simulink model "model1"  (R2024b)
settings: Solver=VariableStepAuto  StartTime=0.0  StopTime=10.0  RelTol=1e-3
values from neighbouring files (symbols this model uses):
  A = [1,2;-3,-4]    [design_AL.m]    (also in run1.m = [[0,1;0,-B/M],zeros(2,2);zeros(2,2),[0,1;0,-Br/J]]; run_p.m; test.m = -1; test2.m = -1)
  Bw = [1;1]    [design_AL.m]    (also in run1.m = zeros(5,1); run_p.m; test.m = 1; test2.m = 1)
  C = [2,1;4,2]    [design_AL.m]    (also in run1.m = [1,0,0,0;0,1,0,0;0,1,0,0;0,0,1,0;0,0,0,1]; run_p.m; test.m = [1;2]; test2.m = [1;2])
  Dw = [1;1]    [design_AL.m]    (also in run1.m = [1;1;1;1;1]; run_p.m; test.m = [1;2]; test2.m = [1;2]*1+[2;-1]*1)
  L = P \ Y    [run_p.m]    (also in test.m = [1,1]; test2.m = inv(P)*Y; test3.m = inv(P)*Y; test4.m = sym('x',[n,p]))
  Lmbda = [x1val,1]    [test2.m]
  Pival = eye(p)-C*pinv(C'*C)*C'    [test.m]    (also in test2.m; test3.m; test4.m)
settings Model: Creator=mehmetcanevi  LastModifiedBy=Mehmet

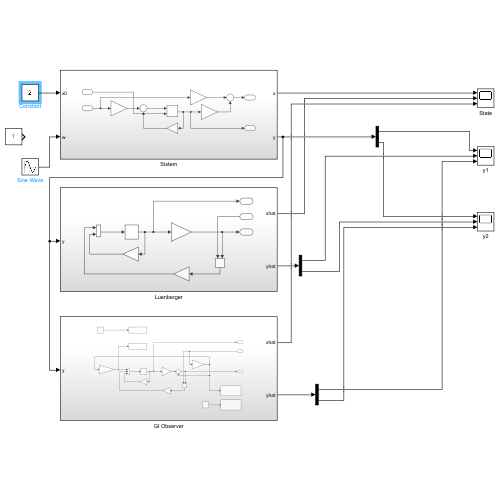
[thumbnail: Simulink's stored preview of the top-level diagram]
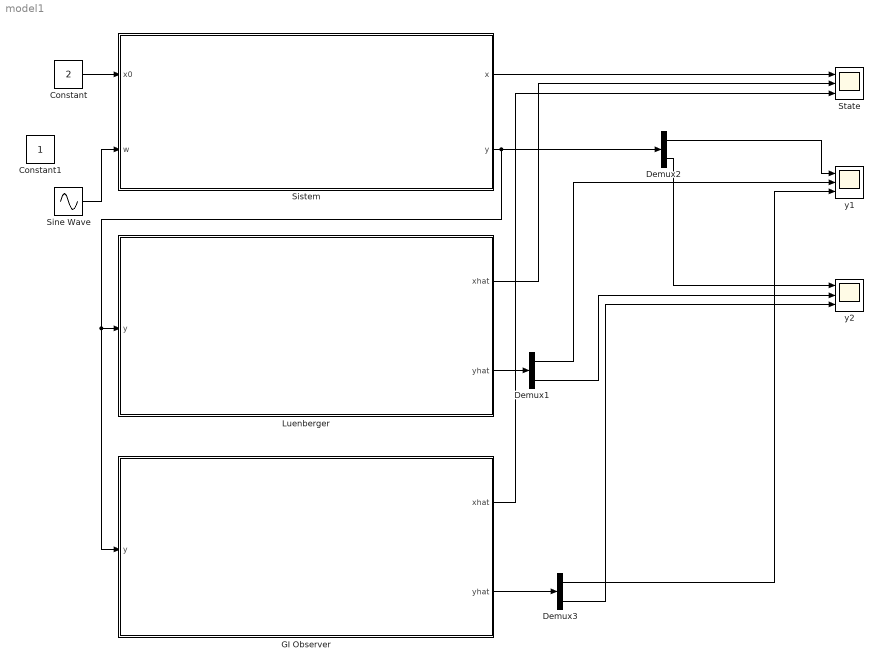
== system model1 ==
  Constant : Constant  Value=2
  Constant1 : Constant
  Demux1 : Demux  Outputs=2
  Demux2 : Demux  Outputs=2
  Demux3 : Demux  Outputs=2
  GI Observer : Subsystem
  Luenberger : Subsystem
  Sine Wave : Sin  SampleTime=0
  Sistem : Subsystem
  State : Scope  NumInputPorts=3
  y1 : Scope  NumInputPorts=3
  y2 : Scope  NumInputPorts=3
  wires:
  GI Observer/2(yhat) -> Demux3/1
  Constant/1 -> Sistem/1(x0)
  Sine Wave/1 -> Sistem/2(w)
  Sistem/1(x) -> State/1
  Sistem/2(y) -> Luenberger/1(y), GI Observer/1(y), Demux2/1
  Luenberger/1(xhat) -> State/2
  GI Observer/1(xhat) -> State/3
  Demux2/1 -> y1/1
  Demux2/2 -> y2/1
  Luenberger/2(yhat) -> Demux1/1
  Demux1/1 -> y1/2
  Demux1/2 -> y2/2
  Demux3/1 -> y1/3
  Demux3/2 -> y2/3

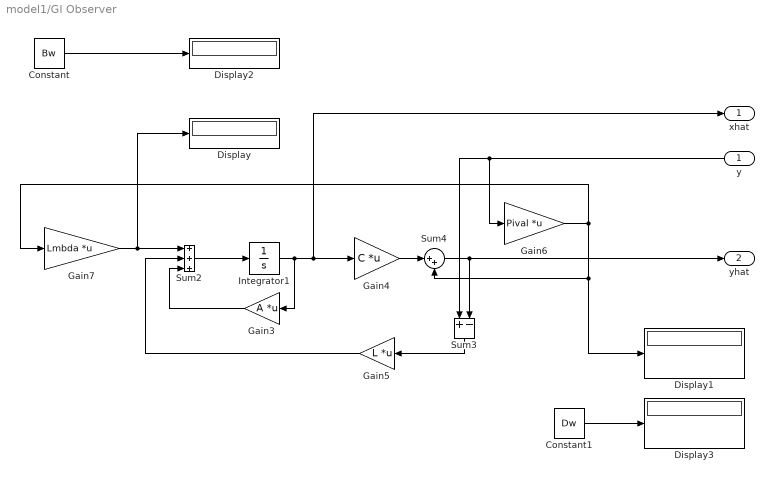
== system model1/GI Observer ==
  y : Inport
  Constant : Constant  Value=Bw
  Constant1 : Constant  Value=Dw
  Display{,1..3} (4 alike) : Display
  Gain3 : Gain  Gain=A  Multiplication=Matrix(K*u)
  Gain4 : Gain  Gain=C  Multiplication=Matrix(K*u)
  Gain5 : Gain  Gain=L  Multiplication=Matrix(K*u)
  Gain6 : Gain  Gain=Pival  Multiplication=Matrix(K*u)
  Gain7 : Gain  Gain=Lmbda  Multiplication=Matrix(K*u)
  Integrator1 : Integrator
  Sum2 : Sum  Inputs=+++
  Sum3 : Sum  Inputs=+-
  Sum4 : Sum  Inputs=|++
  xhat : Outport
  yhat : Outport  Port=2
  wires:
  Integrator1/1 -> xhat/1, Gain4/1, Gain3/1
  Sum2/1 -> Integrator1/1
  Gain6/1 -> Display1/1, Sum4/2, Gain7/1
  Gain7/1 -> Display/1, Sum2/1
  Sum3/1 -> Gain5/1
  Gain3/1 -> Sum2/3
  y/1 -> Sum3/1, Gain6/1
  Gain5/1 -> Sum2/2
  Gain4/1 -> Sum4/1
  Sum4/1 -> Sum3/2, yhat/1
  Constant/1 -> Display2/1
  Constant1/1 -> Display3/1

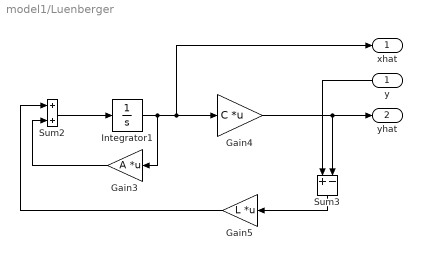
== system model1/Luenberger ==
  y : Inport
  Gain3 : Gain  Gain=A  Multiplication=Matrix(K*u)
  Gain4 : Gain  Gain=C  Multiplication=Matrix(K*u)
  Gain5 : Gain  Gain=L  Multiplication=Matrix(K*u)
  Integrator1 : Integrator
  Sum2 : Sum
  Sum3 : Sum  Inputs=+-
  xhat : Outport
  yhat : Outport  Port=2
  wires:
  Gain5/1 -> Sum2/1
  y/1 -> Sum3/1
  Gain3/1 -> Sum2/2
  Sum3/1 -> Gain5/1
  Gain4/1 -> Sum3/2, yhat/1
  Sum2/1 -> Integrator1/1
  Integrator1/1 -> Gain3/1, Gain4/1, xhat/1

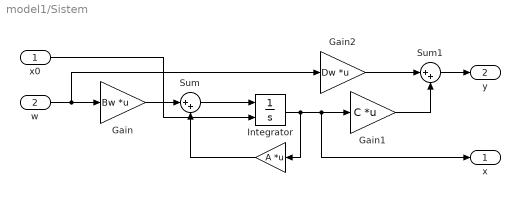
== system model1/Sistem ==
  x0 : Inport
  w : Inport  Port=2
  " " : Gain  Gain=A  Multiplication=Matrix(K*u)
  Gain : Gain  Gain=Bw  Multiplication=Matrix(K*u)
  Gain1 : Gain  Gain=C  Multiplication=Matrix(K*u)
  Gain2 : Gain  Gain=Dw  Multiplication=Matrix(K*u)
  Integrator : Integrator  InitialConditionSource=external
  Sum : Sum  Inputs=|++
  Sum1 : Sum  Inputs=|++
  x : Outport
  y : Outport  Port=2
  wires:
  Gain/1 -> Sum/1
  w/1 -> Gain2/1, Gain/1
  " "/1 -> Sum/2
  Gain2/1 -> Sum1/1
  Integrator/1 -> x/1, Gain1/1, " "/1
  Gain1/1 -> Sum1/2
  Sum1/1 -> y/1
  Sum/1 -> Integrator/1
  x0/1 -> Integrator/2
